simulink model "Model_3rdPoint_Relay"  (R2023b)
settings: Solver=VariableStepAuto  StartTime=0.0  StopTime=H  RelTol=1e-3
values from neighbouring files (symbols this model uses):
  C_f = c_f*m_f    (= 360000)    [init.m]
  C_f_2 = c_f_2*m_f_2    (= 360000)    [init.m]
  C_f_3 = c_f_3*m_f_3    (= 240000)    [init.m]
  C_f_4 = c_f_4*m_f_4    (= 480000)    [init.m]
  k_fc = barK_fc*s_c    (= 570)    [init.m]
  q_s = barK_fc * a    (= 5.529)    [init.m]
  q_star = 5000    [init.m]
  theta0_f = 280    [init.m]
  Ts = 5    [init.m]
  var_wf = 1    [init.m]
settings Model: Creator=adil2  LastModifiedBy=adil2
settings DataIOCC: ReturnWorkspaceOutputs=off

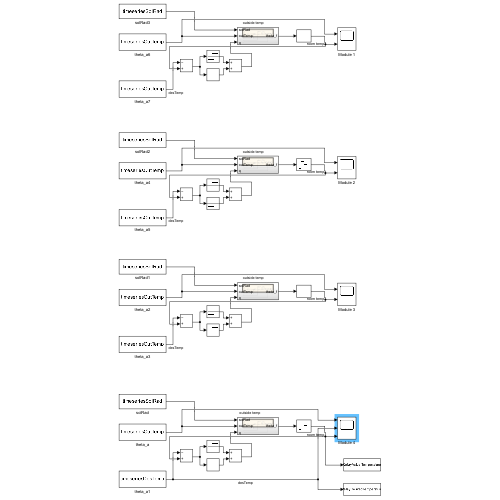
[thumbnail: Simulink's stored preview of the top-level diagram]
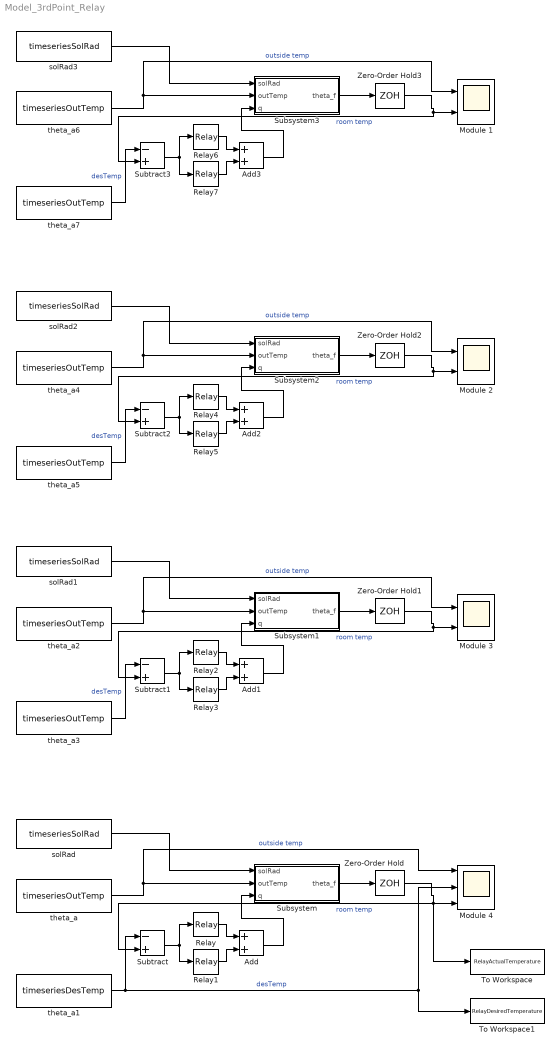
== system Model_3rdPoint_Relay ==
  Add{,1..3} (4 alike) : Sum
  Module 1 : Scope  NumInputPorts=2
  Module 2 : Scope  NumInputPorts=2
  Module 3 : Scope  NumInputPorts=2
  Module 4 : Scope  NumInputPorts=3
  Relay{,2,4,6} (4 alike) : Relay  OnSwitchValue=1  OffSwitchValue=1  OnOutputValue=-q_star  OffOutputValue=q_star
  Relay{1,3,5,7} (4 alike) : Relay  OnSwitchValue=-1  OffSwitchValue=-1  OnOutputValue=-q_star/2  OffOutputValue=q_star/2
  Subsystem : Subsystem
  Subsystem1 : Subsystem
  Subsystem2 : Subsystem
  Subsystem3 : Subsystem
  Subtract{,1..3} (4 alike) : Sum  Inputs=-+
  To Workspace : ToWorkspace  VariableName=RelayActualTemperature  SampleTime=-1
  To Workspace1 : ToWorkspace  VariableName=RelayDesiredTemperature  SampleTime=-1
  Zero-Order Hold{,1..3} (4 alike) : ZeroOrderHold  SampleTime=Ts
  solRad{,1..3} (4 alike) : FromWorkspace  VariableName=timeseriesSolRad
  theta_a{,2..7} (7 alike) : FromWorkspace  VariableName=timeseriesOutTemp  SampleTime=Ts
  theta_a1 : FromWorkspace  VariableName=timeseriesDesTemp  SampleTime=Ts
  wires:
  theta_a1/1 -> Subtract/1, Module 4/2, To Workspace1/1  "desTemp"
  Zero-Order Hold/1 -> To Workspace/1, Subtract/2, Module 4/3  "room temp"
  Subtract/1 -> Relay1/1, Relay/1
  theta_a/1 -> Subsystem/2(outTemp), Module 4/1  "outside temp"
  Subsystem/1(theta_f) -> Zero-Order Hold/1
  solRad/1 -> Subsystem/1(solRad)
  Relay/1 -> Add/1
  Relay1/1 -> Add/2
  Add/1 -> Subsystem/3(q)
  Relay3/1 -> Add1/2
  solRad1/1 -> Subsystem1/1(solRad)
  Subsystem1/1(theta_f) -> Zero-Order Hold1/1
  theta_a2/1 -> Subsystem1/2(outTemp), Module 3/1  "outside temp"
  theta_a3/1 -> Subtract1/1  "desTemp"
  Zero-Order Hold1/1 -> Subtract1/2, Module 3/2  "room temp"
  Subtract1/1 -> Relay3/1, Relay2/1
  Add1/1 -> Subsystem1/3(q)
  Relay2/1 -> Add1/1
  Relay4/1 -> Add2/1
  Add2/1 -> Subsystem2/3(q)
  Subtract2/1 -> Relay5/1, Relay4/1
  theta_a4/1 -> Subsystem2/2(outTemp), Module 2/1  "outside temp"
  Zero-Order Hold2/1 -> Subtract2/2, Module 2/2  "room temp"
  Subsystem2/1(theta_f) -> Zero-Order Hold2/1
  Relay5/1 -> Add2/2
  solRad2/1 -> Subsystem2/1(solRad)
  theta_a5/1 -> Subtract2/1  "desTemp"
  theta_a6/1 -> Subsystem3/2(outTemp), Module 1/1  "outside temp"
  solRad3/1 -> Subsystem3/1(solRad)
  Zero-Order Hold3/1 -> Subtract3/2, Module 1/2  "room temp"
  Subsystem3/1(theta_f) -> Zero-Order Hold3/1
  theta_a7/1 -> Subtract3/1  "desTemp"
  Relay7/1 -> Add3/2
  Subtract3/1 -> Relay7/1, Relay6/1
  Add3/1 -> Subsystem3/3(q)
  Relay6/1 -> Add3/1

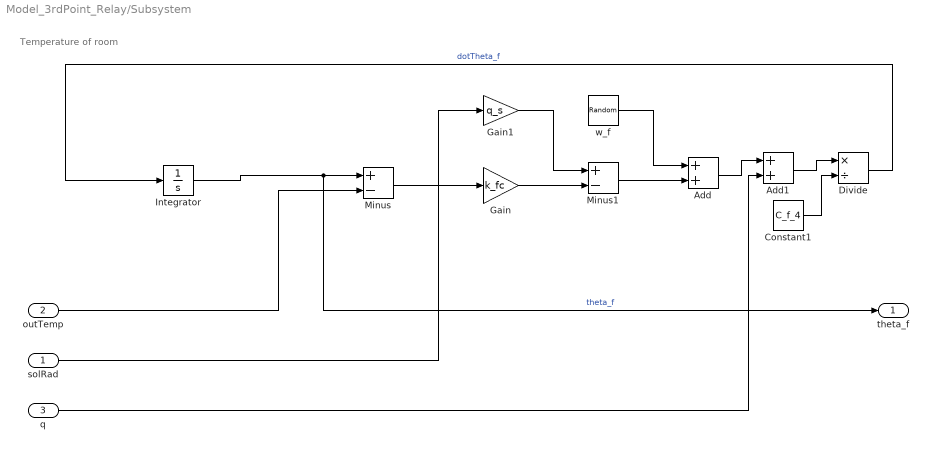
== system Model_3rdPoint_Relay/Subsystem ==
  note: Temperature of room
  solRad : Inport
  outTemp : Inport  Port=2
  q : Inport  Port=3
  Add : Sum
  Add1 : Sum
  Constant1 : Constant  Value=C_f_4
  Divide : Product  Inputs=*/
  Gain : Gain  Gain=k_fc
  Gain1 : Gain  Gain=q_s
  Integrator : Integrator  InitialCondition=theta0_f
  Minus : Sum  Inputs=+-
  Minus1 : Sum  Inputs=+-
  w_f : RandomNumber  Variance=var_wf  SampleTime=Ts
  theta_f : Outport
  wires:
  outTemp/1 -> Minus/2
  Integrator/1 -> theta_f/1, Minus/1  "theta_f"
  Minus/1 -> Gain/1
  Constant1/1 -> Divide/2
  Divide/1 -> Integrator/1  "dotTheta_f"
  Gain/1 -> Minus1/2
  Minus1/1 -> Add/2
  w_f/1 -> Add/1
  solRad/1 -> Gain1/1
  Gain1/1 -> Minus1/1
  Add1/1 -> Divide/1
  Add/1 -> Add1/1
  q/1 -> Add1/2

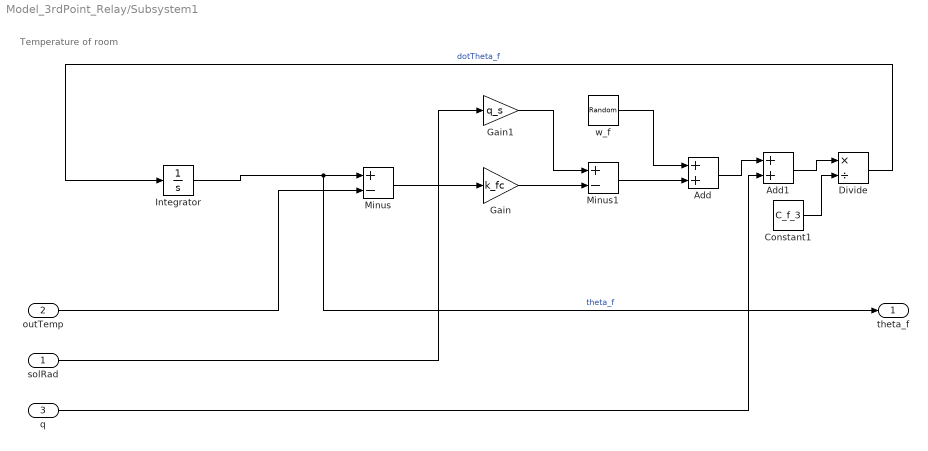
== system Model_3rdPoint_Relay/Subsystem1 ==
  note: Temperature of room
  solRad : Inport
  outTemp : Inport  Port=2
  q : Inport  Port=3
  Add : Sum
  Add1 : Sum
  Constant1 : Constant  Value=C_f_3
  Divide : Product  Inputs=*/
  Gain : Gain  Gain=k_fc
  Gain1 : Gain  Gain=q_s
  Integrator : Integrator  InitialCondition=theta0_f
  Minus : Sum  Inputs=+-
  Minus1 : Sum  Inputs=+-
  w_f : RandomNumber  Variance=var_wf  SampleTime=Ts
  theta_f : Outport
  wires:
  outTemp/1 -> Minus/2
  Integrator/1 -> theta_f/1, Minus/1  "theta_f"
  Minus/1 -> Gain/1
  Constant1/1 -> Divide/2
  Divide/1 -> Integrator/1  "dotTheta_f"
  Gain/1 -> Minus1/2
  Minus1/1 -> Add/2
  w_f/1 -> Add/1
  solRad/1 -> Gain1/1
  Gain1/1 -> Minus1/1
  Add1/1 -> Divide/1
  Add/1 -> Add1/1
  q/1 -> Add1/2

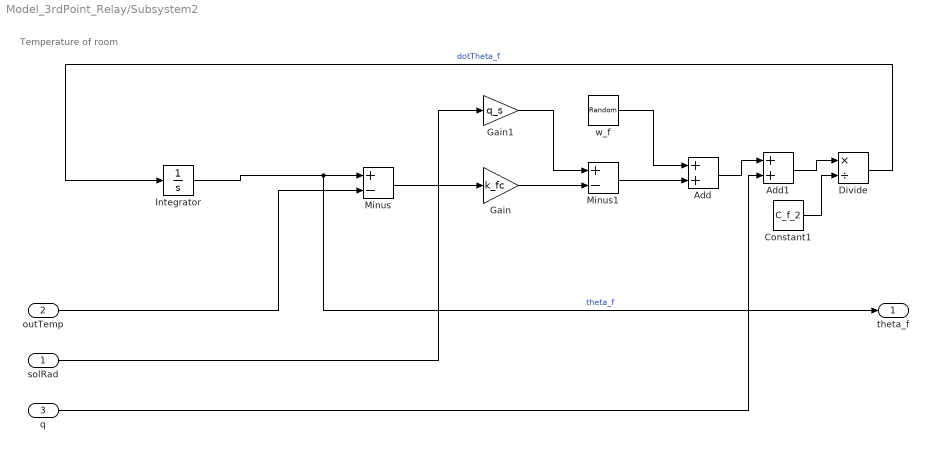
== system Model_3rdPoint_Relay/Subsystem2 ==
  note: Temperature of room
  solRad : Inport
  outTemp : Inport  Port=2
  q : Inport  Port=3
  Add : Sum
  Add1 : Sum
  Constant1 : Constant  Value=C_f_2
  Divide : Product  Inputs=*/
  Gain : Gain  Gain=k_fc
  Gain1 : Gain  Gain=q_s
  Integrator : Integrator  InitialCondition=theta0_f
  Minus : Sum  Inputs=+-
  Minus1 : Sum  Inputs=+-
  w_f : RandomNumber  Variance=var_wf  SampleTime=Ts
  theta_f : Outport
  wires:
  outTemp/1 -> Minus/2
  Integrator/1 -> theta_f/1, Minus/1  "theta_f"
  Minus/1 -> Gain/1
  Constant1/1 -> Divide/2
  Divide/1 -> Integrator/1  "dotTheta_f"
  Gain/1 -> Minus1/2
  Minus1/1 -> Add/2
  w_f/1 -> Add/1
  solRad/1 -> Gain1/1
  Gain1/1 -> Minus1/1
  Add1/1 -> Divide/1
  Add/1 -> Add1/1
  q/1 -> Add1/2

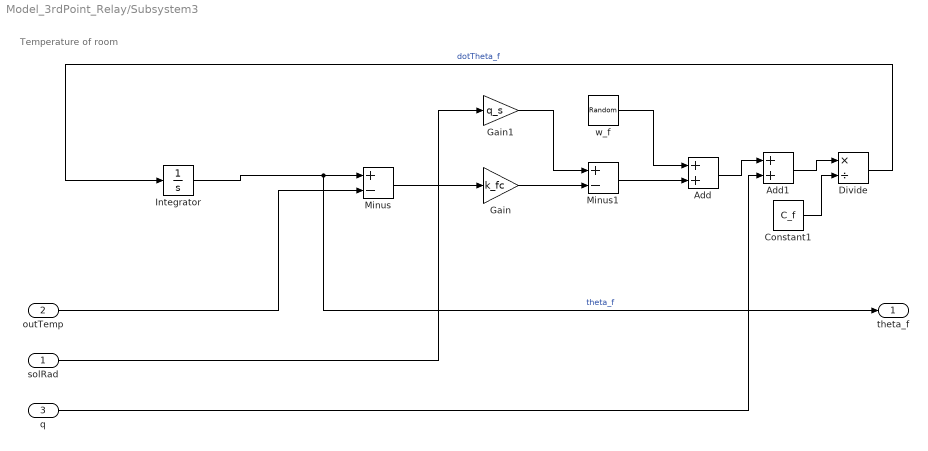
== system Model_3rdPoint_Relay/Subsystem3 ==
  note: Temperature of room
  solRad : Inport
  outTemp : Inport  Port=2
  q : Inport  Port=3
  Add : Sum
  Add1 : Sum
  Constant1 : Constant  Value=C_f
  Divide : Product  Inputs=*/
  Gain : Gain  Gain=k_fc
  Gain1 : Gain  Gain=q_s
  Integrator : Integrator  InitialCondition=theta0_f
  Minus : Sum  Inputs=+-
  Minus1 : Sum  Inputs=+-
  w_f : RandomNumber  Variance=var_wf  SampleTime=Ts
  theta_f : Outport
  wires:
  outTemp/1 -> Minus/2
  Integrator/1 -> theta_f/1, Minus/1  "theta_f"
  Minus/1 -> Gain/1
  Constant1/1 -> Divide/2
  Divide/1 -> Integrator/1  "dotTheta_f"
  Gain/1 -> Minus1/2
  Minus1/1 -> Add/2
  w_f/1 -> Add/1
  solRad/1 -> Gain1/1
  Gain1/1 -> Minus1/1
  Add1/1 -> Divide/1
  Add/1 -> Add1/1
  q/1 -> Add1/2
